simulink model "admittance_controller_quat"  (R2021b)
settings: Solver=VariableStepAuto  StartTime=0.0  StopTime=10.0  RelTol=1e-3
values from neighbouring files (symbols this model uses):
  dphi_cd0 = [0 0 0]'    [admittance_controller.m]    (also in sim_admittance_controller.m; simulation_admittance_controller.m)
  dw_d = [0 0 0]'    [admittance_controller.m]
  h_0e = [f ; mu]    [admittance_controller.m]    (also in sim_admittance_controller.m = [; simulation_admittance_controller.m = timeseries(data, t))
  Kd = eye(3)*kd    [admittance_controller.m]    (also in sim_admittance_controller.m; sim_invdyn.m = eye(3)*50; simulation_admittance_controller.m = eye(3) * 4; simulation_invdyn.m = eye(3)*50)
  Kp = eye(3)*kp    [admittance_controller.m]    (also in sim_admittance_controller.m; sim_invdyn.m = eye(3)*200; simulation_admittance_controller.m = eye(3) * 16; simulation_invdyn.m = eye(3)*200)
  Md = eye(3)*md    [admittance_controller.m]    (also in sim_admittance_controller.m; simulation_admittance_controller.m = eye(3) * 1)
  phi_cd0 = [0 0 0]'    [admittance_controller.m]    (also in sim_admittance_controller.m; simulation_admittance_controller.m)
  q_d = quaternion(phi_d', "euler", "XYZ", "frame").compact()    [admittance_controller.m]    (also in quat_tf_test.m = UnitQuaternion(eta_d, eps_d); sim_admittance_controller.m = rotm2quat(R_ds); sim_invdyn.m = ref(:, 1); simulation_admittance_controller.m = timeseries(data, t))
  T_d = trvec2tform(p_d') * eul2tform(phi_d', "XYZ")    [admittance_controller.m]    (also in sim_admittance_controller.m = trvec2tform([0.5 0.0 0.2]) * eul2tform([-pi/4 1 pi/4], "XYZ"; simulation_admittance_controller.m = trvec2tform([0.6    0 0.4]) * eul2tform([-1.2 1 -1.2], "XYZ")
  w_d = vel(1:3, :)'    [admittance_controller.m]
undefined symbols (not defined in the file or in its folder): compact
settings Model: Creator=Martin  LastModifiedBy=Martin

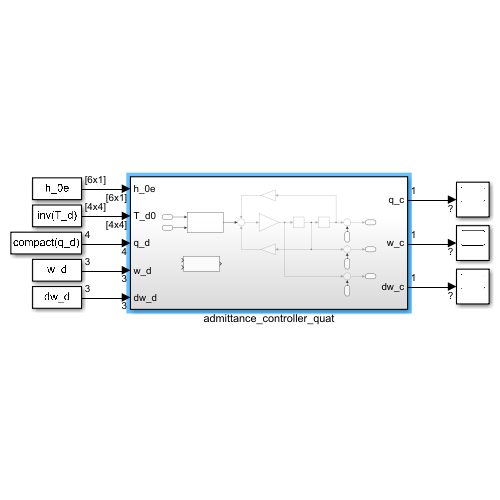
[thumbnail: Simulink's stored preview of the top-level diagram]
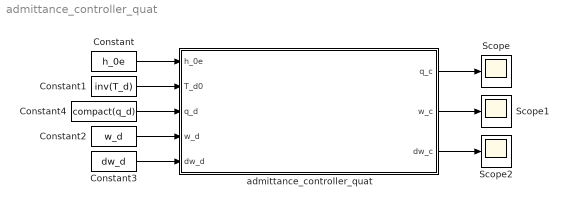
== system admittance_controller_quat ==
  Constant : Constant  Value=h_0e  VectorParams1D=off
  Constant1 : Constant  Value=inv(T_d)
  Constant2 : Constant  Value=w_d
  Constant3 : Constant  Value=dw_d
  Constant4 : Constant  Value=compact(q_d)
  Scope : Scope
  Scope1 : Scope
  Scope2 : Scope
  admittance_controller_quat : Subsystem
  wires:
  Constant/1 -> admittance_controller_quat/1(h_0e)
  Constant2/1 -> admittance_controller_quat/4(w_d)
  Constant3/1 -> admittance_controller_quat/5(dw_d)
  admittance_controller_quat/1(q_c) -> Scope/1
  admittance_controller_quat/2(w_c) -> Scope1/1
  admittance_controller_quat/3(dw_c) -> Scope2/1
  Constant4/1 -> admittance_controller_quat/3(q_d)
  Constant1/1 -> admittance_controller_quat/2(T_d0)

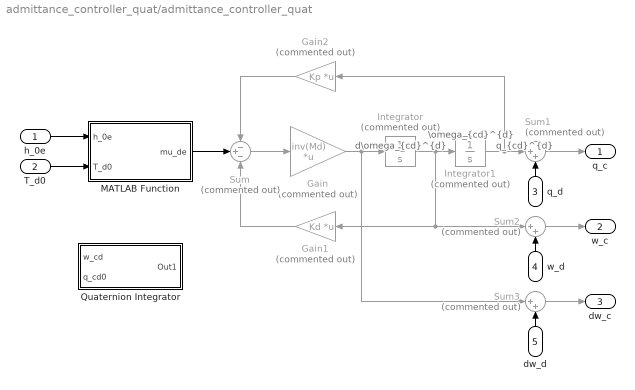
== system admittance_controller_quat/admittance_controller_quat ==
  note: q_{cd}^{d}
  note: \omega_{cd}^{d}
  note: d\omega_{cd}^{d}
  h_0e : Inport
  T_d0 : Inport  Port=2
  q_d : Inport  Port=3
  w_d : Inport  Port=4
  dw_d : Inport  Port=5
  Gain : Gain  Commented=on  Gain=inv(Md)  Multiplication=Matrix(K*u)
  Gain1 : Gain  Commented=on  Gain=Kd  Multiplication=Matrix(K*u)
  Gain2 : Gain  Commented=on  Gain=Kp  Multiplication=Matrix(K*u)
  Integrator : Integrator  Commented=on  InitialCondition=dphi_cd0
  Integrator1 : Integrator  Commented=on  InitialCondition=phi_cd0
  MATLAB Function : MATLAB Function  TreatAsAtomicUnit=on
  Quaternion Integrator : Subsystem
  Sum : Sum  Commented=on  Inputs=-+-
  Sum1 : Sum  Commented=on  Inputs=|++
  Sum2 : Sum  Commented=on  Inputs=|++
  Sum3 : Sum  Commented=on  Inputs=|++
  q_c : Outport
  w_c : Outport  Port=2
  dw_c : Outport  Port=3
  wires:
  Sum2/1 -> w_c/1
  Sum3/1 -> dw_c/1
  Integrator/1 -> Gain1/1, Sum2/1, Integrator1/1
  Integrator1/1 -> Sum1/1, Gain2/1
  w_d/1 -> Sum2/2
  Gain/1 -> Sum3/1, Integrator/1
  dw_d/1 -> Sum3/2
  Sum1/1 -> q_c/1
  Sum/1 -> Gain/1
  Gain2/1 -> Sum/1
  Gain1/1 -> Sum/3
  h_0e/1 -> MATLAB Function/1(h_0e)
  MATLAB Function/1(mu_de) -> Sum/2
  T_d0/1 -> MATLAB Function/2(T_d0)
  q_d/1 -> Sum1/2

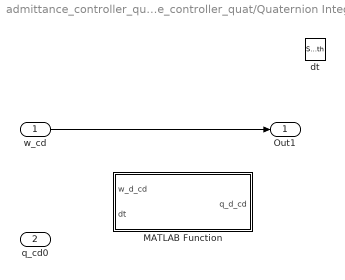
== system admittance_controller_quat/admittance_controller_quat/Quaternion Integrator ==
  w_cd : Inport
  q_cd0 : Inport  Port=2
  MATLAB Function : MATLAB Function  TreatAsAtomicUnit=on
  dt : SampleTimeMath  TsampMathOp=Ts Only
  Out1 : Outport
  wires:
  w_cd/1 -> Out1/1

== matlab function admittance_controller_quat/MATLAB Function ==
  data: h_0e input; mu_de output; T_d0 input
function mu_de = wrench_tf(h_0e, T_d0)

    % given end-effector wrench h_0e in base frame
    % transform such that given in desired frame, h_de

    R_d0 = tform2rotm(T_d0);
    t_d0 = tform2trvec(T_d0);
    % Ad   = [R_d0 0 ; skew(t_d0) * R_d0 R_d0];

    mu_de = [skew(t_d0) * R_d0 R_d0] * h_0e; % only for moment

end

== matlab function admittance_controller_quat/Quaternion Integrator/MATLAB Function ==
  data: w_d_cd input; q_d_cd output; dt input
function q_d_cd = fcn(w_d_cd, dt)

end
